simulink model "implementacao_em_blocos"  (R2013a)
settings: Solver=ode45  StartTime=0.0  StopTime=500  RelTol=1e-3
libraries: aerolibutil x4, vrlib x4, aerolibtransform2 x2, dspmtrx3 x1
settings Model: Creator=Daniel  LastModifiedBy=Daniel

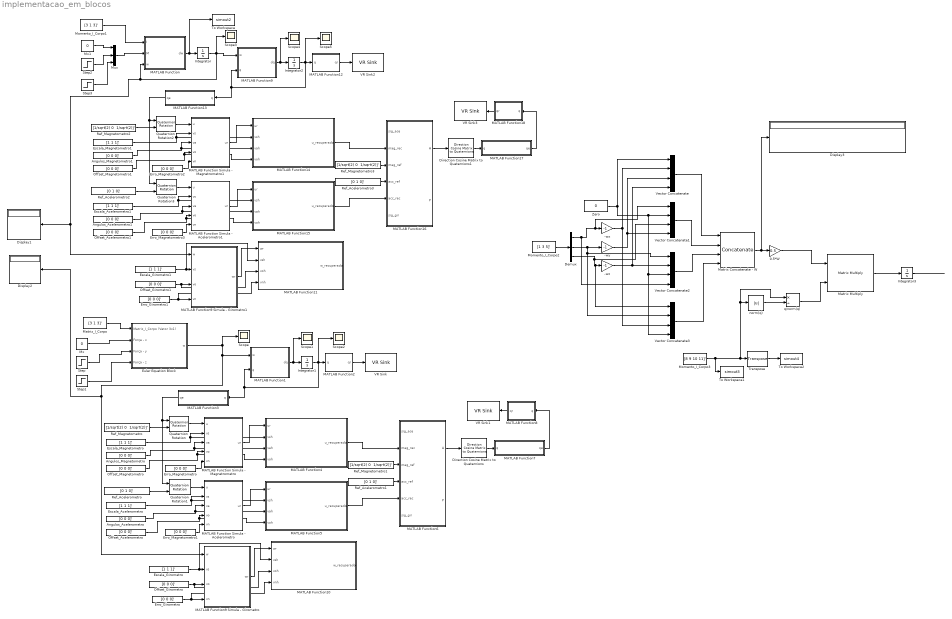
== system implementacao_em_blocos ==
  -wx : Gain  Gain=-1
  -wy : Gain  Gain=-1
  -wz : Gain  Gain=-1
  0.5*W : Gain  Gain=0.5
  Angulos_Acelerometro : Constant  Value=[0 0 0]'
  Angulos_Acelerometro1 : Constant  Value=[0 0 0]'
  Angulos_Magnetometro : Constant  Value=[0 0 0]'
  Angulos_Magnetometro1 : Constant  Value=[0 0 0]'
  Demux : Demux  Outputs=3
  Direction Cosine Matrix to Quaternions : aerolibtransform2/Direction Cosine Matrix  to Quaternions
  Direction Cosine Matrix to Quaternions1 : aerolibtransform2/Direction Cosine Matrix  to Quaternions
  Display1 : Display
  Display2 : Display
  Display3 : Display
  Erro_Girometro : Constant  Value=[0 0 0]'
  Erro_Girometro1 : Constant  Value=[0 0 0]'
  Erro_Magnetometro{,1..3} (4 alike) : Constant  Value=[0 0 0]'
  Escala_Acelerometro : Constant  Value=[1 1 1]'
  Escala_Acelerometro1 : Constant  Value=[1 1 1]'
  Escala_Girometro : Constant  Value=[1 1 1]'
  Escala_Girometro1 : Constant  Value=[1 1 1]'
  Escala_Magnetometro : Constant  Value=[1 1 1]'
  Escala_Magnetometro1 : Constant  Value=[1 1 1]'
  Euler Equation Block : Subsystem
  Integrator : Integrator  InitialCondition=[0 0 0]
  Integrator1 : Integrator  InitialCondition=[1 0 0 0]
  Integrator2 : Integrator  InitialCondition=[1 0 0 0]
  Integrator3 : Integrator  InitialCondition=[1 0 0 0]'
  MATLAB Function : MATLAB Function  TreatAsAtomicUnit=on
  MATLAB Function Simula - Acelerometro : MATLAB Function  TreatAsAtomicUnit=on
  MATLAB Function Simula - Acelerometro1 : MATLAB Function  TreatAsAtomicUnit=on
  MATLAB Function Simula - Magnetrometro : MATLAB Function  TreatAsAtomicUnit=on
  MATLAB Function Simula - Magnetrometro1 : MATLAB Function  TreatAsAtomicUnit=on
  MATLAB Function1 : MATLAB Function  TreatAsAtomicUnit=on
  MATLAB Function10 : MATLAB Function  TreatAsAtomicUnit=on
  MATLAB Function11 : MATLAB Function  TreatAsAtomicUnit=on
  MATLAB Function12 : MATLAB Function  TreatAsAtomicUnit=on
  MATLAB Function13 : MATLAB Function  TreatAsAtomicUnit=on
  MATLAB Function14 : MATLAB Function  TreatAsAtomicUnit=on
  MATLAB Function15 : MATLAB Function  TreatAsAtomicUnit=on
  MATLAB Function16 : MATLAB Function  TreatAsAtomicUnit=on
  MATLAB Function17 : MATLAB Function  TreatAsAtomicUnit=on
  MATLAB Function18 : MATLAB Function  TreatAsAtomicUnit=on
  MATLAB Function2 : MATLAB Function  TreatAsAtomicUnit=on
  MATLAB Function3 : MATLAB Function  TreatAsAtomicUnit=on
  MATLAB Function4 : MATLAB Function  TreatAsAtomicUnit=on
  MATLAB Function5 : MATLAB Function  TreatAsAtomicUnit=on
  MATLAB Function6 : MATLAB Function  TreatAsAtomicUnit=on
  MATLAB Function7 : MATLAB Function  TreatAsAtomicUnit=on
  MATLAB Function8 : MATLAB Function  TreatAsAtomicUnit=on
  MATLAB Function9 : MATLAB Function  TreatAsAtomicUnit=on
  MATLAB Function9 Simula - Girometro : MATLAB Function  TreatAsAtomicUnit=on
  MATLAB Function9 Simula - Girometro1 : MATLAB Function  TreatAsAtomicUnit=on
  Matrix Concatenate - W : Concatenate  NumInputs=4  Mode=Multidimensional array
  Matrix Multiply : Product  Multiplication=Matrix(*)
  Matriz_I_Corpo : Constant  Value=[3 1 3]'  VectorParams1D=off
  Momento_I_Corpo1 : Constant  Value=[3 1 3]'
  Momento_I_Corpo2 : Constant  Value=[1 3 5]'
  Momento_I_Corpo3 : Constant  Value=[8 9 10 11]'  VectorParams1D=off
  Mux : Mux  Inputs=3
  Mx : Constant  Value=0
  Mx1 : Constant  Value=0
  Offset_Acelerometro : Constant  Value=[0 0 0]'
  Offset_Acelerometro1 : Constant  Value=[0 0 0]'
  Offset_Girometro : Constant  Value=[0 0 0]'
  Offset_Girometro1 : Constant  Value=[0 0 0]'
  Offset_Magnetometro : Constant  Value=[0 0 0]'
  Offset_Magnetometro1 : Constant  Value=[0 0 0]'
  Quaternion Rotation{,1..3} (4 alike) : aerolibutil/Quaternion Rotation
  Ref_Acelerometro{,1..3} (4 alike) : Constant  Value=[0 1 0]'
  Ref_Magnetometro{,1..3} (4 alike) : Constant  Value="[1/sqrt(2) 0  1/sqrt(2)]'"
  Scope{,1..5} (6 alike) : Scope
      Scope2 settings: SaveName=ScopeData2
      Scope3 settings: SaveName=ScopeData3
      Scope4 settings: SaveName=ScopeData4
      Scope5 settings: SaveName=ScopeData5
  Step : Step  Before=1  After=0  SampleTime=0
  Step1 : Step  Before=.5  After=0  SampleTime=0
  Step2 : Step  Before=1  After=0  SampleTime=0
  Step3 : Step  Before=.5  After=0  SampleTime=0
  To Workspace : ToWorkspace  VariableName=simout2  SampleTime=-1
  To Workspace1 : ToWorkspace  VariableName=simout3  SampleTime=-1
  To Workspace2 : ToWorkspace  VariableName=simout4  SampleTime=-1
  Transpose : dspmtrx3/Transpose  Hermitian=off  overflowFlag=off
  VR Sink : vrlib/VR Sink  InstantiateOnLoad=on  SampleTime=.1  ViewEnable=on  RemoteChange=off  RemoteView=off  FieldsWritten=H.rotation.4.1.1.double  WorldFileName=C:\Users\Daniel\Desktop\TCC Daniel\Arquivos WRL\cilindro_bloco3.wrl  AutoView=off  VideoDimensions=[]  AllowVariableSize=off
  VR Sink1 : vrlib/VR Sink  InstantiateOnLoad=on  SampleTime=.1  ViewEnable=on  RemoteChange=off  RemoteView=off  FieldsWritten=H.rotation.4.1.1.double  WorldFileName=C:\Users\Daniel\Desktop\TCC Daniel\Arquivos WRL\cilindro_bloco4.wrl  AutoView=off  VideoDimensions=[]  AllowVariableSize=off
  VR Sink2 : vrlib/VR Sink  InstantiateOnLoad=on  SampleTime=.1  ViewEnable=on  RemoteChange=off  RemoteView=off  FieldsWritten=H.rotation.4.1.1.double  WorldFileName=C:\Users\Daniel\Desktop\TCC Daniel\Arquivos WRL\cilindro_bloco1.wrl  AutoView=off  VideoDimensions=[]  AllowVariableSize=off
  VR Sink3 : vrlib/VR Sink  InstantiateOnLoad=on  SampleTime=.1  ViewEnable=on  RemoteChange=off  RemoteView=off  FieldsWritten=H.rotation.4.1.1.double  WorldFileName=C:\Users\Daniel\Desktop\TCC Daniel\Arquivos WRL\cilindro_bloco2.wrl  AutoView=off  VideoDimensions=[]  AllowVariableSize=off
  Vector Concatenate{,1..3} (4 alike) : Concatenate  NumInputs=4  Mode=Multidimensional array  ConcatenateDimension=2
  Zero : Constant  Value=0
  norm(q) : Abs
  q/norm(q) : Product  Inputs=*/
  wires:
  Mux/1 -> MATLAB Function/2(M)
  MATLAB Function/1(dw) -> To Workspace/1, Integrator/1
  MATLAB Function1/1(dq) -> Integrator1/1, Scope1/1
  Integrator1/1 -> MATLAB Function3/1(q), MATLAB Function1/2(q), Scope2/1, MATLAB Function2/1(q)
  MATLAB Function2/1(qr) -> VR Sink/1
  Quaternion Rotation/1 -> MATLAB Function Simula - Magnetrometro/1(u)
  Quaternion Rotation1/1 -> MATLAB Function Simula - Acelerometro/1(u)
  MATLAB Function3/1(qe) -> Quaternion Rotation/1, Quaternion Rotation1/1
  Ref_Magnetometro/1 -> Quaternion Rotation/2
  Ref_Acelerometro/1 -> Quaternion Rotation1/2
  Erro_Magnetometro/1 -> MATLAB Function Simula - Magnetrometro/5(vn)
  Erro_Magnetometro1/1 -> MATLAB Function Simula - Acelerometro/5(vn)
  Offset_Magnetometro/1 -> MATLAB Function Simula - Magnetrometro/4(vo), MATLAB Function4/4(voh)
  Escala_Acelerometro/1 -> MATLAB Function Simula - Acelerometro/2(vs), MATLAB Function5/2(vsh)
  Angulos_Acelerometro/1 -> MATLAB Function Simula - Acelerometro/3(va), MATLAB Function5/3(vah)
  Offset_Acelerometro/1 -> MATLAB Function Simula - Acelerometro/4(vo), MATLAB Function5/4(voh)
  MATLAB Function Simula - Magnetrometro/1(ur) -> MATLAB Function4/1(ur)
  MATLAB Function Simula - Acelerometro/1(ur) -> MATLAB Function5/1(ur)
  Escala_Magnetometro/1 -> MATLAB Function Simula - Magnetrometro/2(vs), MATLAB Function4/2(vsh)
  Angulos_Magnetometro/1 -> MATLAB Function Simula - Magnetrometro/3(va), MATLAB Function4/3(vah)
  MATLAB Function5/1(u_recuperado) -> MATLAB Function6/5(acc_rec)
  MATLAB Function4/1(u_recuperado) -> MATLAB Function6/2(mag_rec)
  Ref_Magnetometro1/1 -> MATLAB Function6/3(mag_ref)
  Ref_Acelerometro1/1 -> MATLAB Function6/4(acc_ref)
  MATLAB Function6/1(A) -> Direction Cosine Matrix to Quaternions/1
  MATLAB Function7/1(qe) -> MATLAB Function8/1(q)
  MATLAB Function9 Simula - Girometro/1(wr) -> MATLAB Function10/1(wr)
  Escala_Girometro/1 -> MATLAB Function10/2(vsh), MATLAB Function9 Simula - Girometro/2(vs)
  Offset_Girometro/1 -> MATLAB Function10/3(voh), MATLAB Function9 Simula - Girometro/3(vo)
  Direction Cosine Matrix to Quaternions/1 -> MATLAB Function7/1(q)
  Erro_Girometro/1 -> MATLAB Function10/4(vnh), MATLAB Function9 Simula - Girometro/4(vn)
  MATLAB Function8/1(qr) -> VR Sink1/1
  MATLAB Function9/1(dq) -> Integrator2/1, Scope4/1
  Integrator2/1 -> MATLAB Function13/1(q), MATLAB Function9/2(q), Scope5/1, MATLAB Function12/1(q)
  MATLAB Function12/1(qr) -> VR Sink2/1
  Quaternion Rotation2/1 -> MATLAB Function Simula - Magnetrometro1/1(u)
  Quaternion Rotation3/1 -> MATLAB Function Simula - Acelerometro1/1(u)
  MATLAB Function13/1(qe) -> Quaternion Rotation2/1, Quaternion Rotation3/1
  Ref_Magnetometro2/1 -> Quaternion Rotation2/2
  Ref_Acelerometro2/1 -> Quaternion Rotation3/2
  Erro_Magnetometro2/1 -> MATLAB Function Simula - Magnetrometro1/5(vn)
  Erro_Magnetometro3/1 -> MATLAB Function Simula - Acelerometro1/5(vn)
  Offset_Magnetometro1/1 -> MATLAB Function Simula - Magnetrometro1/4(vo), MATLAB Function14/4(voh)
  Escala_Acelerometro1/1 -> MATLAB Function Simula - Acelerometro1/2(vs), MATLAB Function15/2(vsh)
  Angulos_Acelerometro1/1 -> MATLAB Function Simula - Acelerometro1/3(va), MATLAB Function15/3(vah)
  Offset_Acelerometro1/1 -> MATLAB Function Simula - Acelerometro1/4(vo), MATLAB Function15/4(voh)
  MATLAB Function Simula - Magnetrometro1/1(ur) -> MATLAB Function14/1(ur)
  MATLAB Function Simula - Acelerometro1/1(ur) -> MATLAB Function15/1(ur)
  Escala_Magnetometro1/1 -> MATLAB Function Simula - Magnetrometro1/2(vs), MATLAB Function14/2(vsh)
  Angulos_Magnetometro1/1 -> MATLAB Function Simula - Magnetrometro1/3(va), MATLAB Function14/3(vah)
  MATLAB Function15/1(u_recuperado) -> MATLAB Function16/5(acc_rec)
  MATLAB Function14/1(u_recuperado) -> MATLAB Function16/2(mag_rec)
  Ref_Magnetometro3/1 -> MATLAB Function16/3(mag_ref)
  Ref_Acelerometro3/1 -> MATLAB Function16/4(acc_ref)
  MATLAB Function16/1(A) -> Direction Cosine Matrix to Quaternions1/1
  MATLAB Function17/1(qe) -> MATLAB Function18/1(q)
  MATLAB Function9 Simula - Girometro1/1(wr) -> MATLAB Function11/1(wr)
  Escala_Girometro1/1 -> MATLAB Function11/2(vsh), MATLAB Function9 Simula - Girometro1/2(vs)
  Offset_Girometro1/1 -> MATLAB Function11/3(voh), MATLAB Function9 Simula - Girometro1/3(vo)
  Direction Cosine Matrix to Quaternions1/1 -> MATLAB Function17/1(q)
  Erro_Girometro1/1 -> MATLAB Function11/4(vnh), MATLAB Function9 Simula - Girometro1/4(vn)
  MATLAB Function18/1(qr) -> VR Sink3/1
  Matriz_I_Corpo/1 -> Euler Equation Block/1(Matriz_I_Corpo (Vetor 3x1))
  Mx/1 -> Euler Equation Block/2(Força - x)
  Step/1 -> Euler Equation Block/3(Força - y)
  Step1/1 -> Euler Equation Block/4(Força - z)
  Momento_I_Corpo1/1 -> MATLAB Function/1(I)
  Mx1/1 -> Mux/1
  Step2/1 -> Mux/2
  Step3/1 -> Mux/3
  Integrator/1 -> Scope3/1, MATLAB Function/3(w), Display1/1, MATLAB Function9 Simula - Girometro1/1(w), MATLAB Function9/1(w)
  Euler Equation Block/1(w) -> MATLAB Function9 Simula - Girometro/1(w), Display2/1, MATLAB Function1/1(w), Scope/1
  Momento_I_Corpo3/1 -> To Workspace1/1, Transpose/1, q/norm(q)/1, norm(q)/1
  norm(q)/1 -> q/norm(q)/2
  Demux/3 -> Vector Concatenate3/1, -wz/1, Vector Concatenate1/3
  Demux/2 -> Vector Concatenate3/2, Vector Concatenate2/1, -wy/1
  Demux/1 -> Vector Concatenate2/4, Vector Concatenate1/1, -wx/1
  Zero/1 -> Vector Concatenate3/4, Vector Concatenate2/3, Vector Concatenate1/2, Vector Concatenate/1
  -wx/1 -> Vector Concatenate3/3, Vector Concatenate/2
  -wy/1 -> Vector Concatenate1/4, Vector Concatenate/3
  -wz/1 -> Vector Concatenate2/2, Vector Concatenate/4
  Vector Concatenate/1 -> Matrix Concatenate - W/1
  Vector Concatenate1/1 -> Matrix Concatenate - W/2
  Vector Concatenate2/1 -> Matrix Concatenate - W/3
  Vector Concatenate3/1 -> Matrix Concatenate - W/4
  Matrix Concatenate - W/1 -> 0.5*W/1, Display3/1
  Momento_I_Corpo2/1 -> Demux/1
  q/norm(q)/1 -> Matrix Multiply/2
  0.5*W/1 -> Matrix Multiply/1
  Transpose/1 -> To Workspace2/1
  Matrix Multiply/1 -> Integrator3/1
  Integrator3/1 -> ?

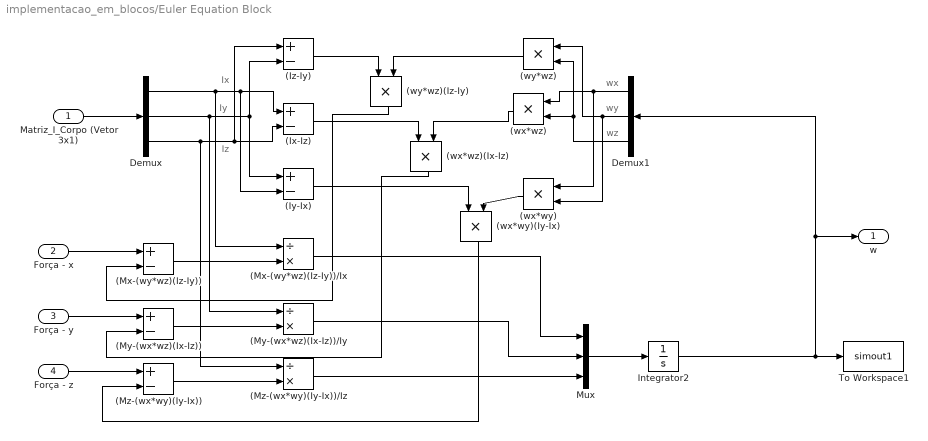
== system implementacao_em_blocos/Euler Equation Block ==
  note: Iz
  note: Iy
  note: Ix
  note: wy
  note: wx
  note: wz
  Matriz_I_Corpo (Vetor 3x1) : Inport
  Força - x : Inport  Port=2
  Força - y : Inport  Port=3
  Força - z : Inport  Port=4
  (Ix-Iz) : Sum  Inputs=+-
  (Iy-Ix) : Sum  Inputs=+-
  (Iz-Iy) : Sum  Inputs=+-
  (Mx-(wy*wz)(Iz-Iy)) : Sum  Inputs=+-
  (Mx-(wy*wz)(Iz-Iy))/Ix : Product  Inputs=/*
  (My-(wx*wz)(Ix-Iz)) : Sum  Inputs=+-
  (My-(wx*wz)(Ix-Iz))/Iy : Product  Inputs=/*
  (Mz-(wx*wy)(Iy-Ix)) : Sum  Inputs=+-
  (Mz-(wx*wy)(Iy-Ix))/Iz : Product  Inputs=/*
  (wx*wy) : Product
  (wx*wy)(Iy-Ix) : Product
  (wx*wz) : Product
  (wx*wz)(Ix-Iz) : Product
  (wy*wz) : Product
  (wy*wz)(Iz-Iy) : Product
  Demux : Demux  Outputs=3
  Demux1 : Demux  Outputs=3
  Integrator2 : Integrator  InitialCondition=[0 0 0]
  Mux : Mux  Inputs=3
  To Workspace1 : ToWorkspace  VariableName=simout1  SampleTime=-1
  w : Outport
  wires:
  (Mz-(wx*wy)(Iy-Ix))/1 -> (Mz-(wx*wy)(Iy-Ix))/Iz/2
  Demux/3 -> (Mz-(wx*wy)(Iy-Ix))/Iz/1, (Iz-Iy)/1, (Ix-Iz)/2
  Força - z/1 -> (Mz-(wx*wy)(Iy-Ix))/1
  (wx*wy)(Iy-Ix)/1 -> (Mz-(wx*wy)(Iy-Ix))/2
  (wy*wz)(Iz-Iy)/1 -> (Mx-(wy*wz)(Iz-Iy))/2
  (My-(wx*wz)(Ix-Iz))/1 -> (My-(wx*wz)(Ix-Iz))/Iy/2
  (My-(wx*wz)(Ix-Iz))/Iy/1 -> Mux/2
  (Iz-Iy)/1 -> (wy*wz)(Iz-Iy)/1
  Demux1/2 -> (wx*wy)/2, (wy*wz)/1
  (Ix-Iz)/1 -> (wx*wz)(Ix-Iz)/1
  (wx*wz)/1 -> (wx*wz)(Ix-Iz)/2
  (wy*wz)/1 -> (wy*wz)(Iz-Iy)/2
  Demux1/1 -> (wx*wy)/1, (wx*wz)/1
  Demux1/3 -> (wy*wz)/2, (wx*wz)/2
  (wx*wy)/1 -> (wx*wy)(Iy-Ix)/2
  (Iy-Ix)/1 -> (wx*wy)(Iy-Ix)/1
  (wx*wz)(Ix-Iz)/1 -> (My-(wx*wz)(Ix-Iz))/2
  Força - x/1 -> (Mx-(wy*wz)(Iz-Iy))/1
  (Mz-(wx*wy)(Iy-Ix))/Iz/1 -> Mux/3
  Demux/1 -> (Mx-(wy*wz)(Iz-Iy))/Ix/1, (Iy-Ix)/2, (Ix-Iz)/1
  Demux/2 -> (My-(wx*wz)(Ix-Iz))/Iy/1, (Iy-Ix)/1, (Iz-Iy)/2
  (Mx-(wy*wz)(Iz-Iy))/1 -> (Mx-(wy*wz)(Iz-Iy))/Ix/2
  Força - y/1 -> (My-(wx*wz)(Ix-Iz))/1
  Matriz_I_Corpo (Vetor 3x1)/1 -> Demux/1
  Mux/1 -> Integrator2/1
  (Mx-(wy*wz)(Iz-Iy))/Ix/1 -> Mux/1
  Integrator2/1 -> To Workspace1/1, Demux1/1, w/1

== matlab function implementacao_em_blocos/MATLAB Function1 ==
  data: w input; dq output; q input
function dq = cinematica(w,q)
%#eml
wx = w(1);
wy = w(2);
wz = w(3);

q = q/norm(q);

qteta = q(1);
qx = q(2);
qy = q(3);
qz = q(4);

W = [0 -wx -wy -wz; wx 0 wz -wy; wy -wz 0 wx; wz wy -wx 0];
%W=[0 wz -wy wx; -wz 0 wx wy; wy -wx 0 wz; -wx -wy -wz 0];
dq=0.5*W*[qteta qx qy qz]';

== matlab function implementacao_em_blocos/MATLAB Function ==
  data: I input; dw output; M input; w input
function dw  = Eq_Euler(I,M,w)
%#eml
wx = w(1);
wy = w(2);
wz = w(3);

Ix = I(1);
Iy = I(2);
Iz = I(3);

Mx = M(1);
My = M(2);
Mz = M(3);

dwx = (Mx - wy*wz*(Iz - Iy))/Ix;
dwy = (My - wx*wz*(Ix - Iz))/Iy;
dwz = (Mz - wx*wy*(Iy - Ix))/Iz;

dw=[dwx dwy dwz];

== matlab function implementacao_em_blocos/MATLAB Function2 ==
  data: q input; qr output
function qr = ajusta_q(q)
%#eml

q = q/(norm(q));
v = [q(2) q(3) q(4)] / norm([q(2) q(3) q(4)]);
ang = acos(q(1))*2;

qr = [v ang];

== matlab function implementacao_em_blocos/MATLAB Function3 ==
  data: q input; qe output
function qe = tira_redundancia(q)
qe = zeros(4,1);
%#eml

if q(1)<0
    qe = -q;
else
    qe = q;
end

== matlab function implementacao_em_blocos/MATLAB Function Simula - Magnetrometro ==
  data: u input; ur output; vs input; va input; vo input; vn input
function ur = triad_model(u,vs,va,vo,vn)
%#eml

rho = va(1);
phi = va(2);
lambda = va(3);

S = diag(vs);
T = [1 0 0; sin(rho) cos(rho) 0;...
    sin(phi)*cos(lambda) sin(lambda)*cos(phi) cos(phi)*cos(lambda)];

ur = S*T*u + vo + vn*randn;

== matlab function implementacao_em_blocos/MATLAB Function Simula - Acelerometro ==
  data: u input; ur output; vs input; va input; vo input; vn input
function ur = triad_model(u,vs,va,vo,vn)
%#eml

rho = va(1);
phi = va(2);
lambda = va(3);

S = diag(vs);
T = [1 0 0; sin(rho) cos(rho) 0;...
    sin(phi)*cos(lambda) sin(lambda)*cos(phi) cos(phi)*cos(lambda)];

ur = S*T*u + vo + vn*randn;

== matlab function implementacao_em_blocos/MATLAB Function4 ==
  data: ur input; u_recuperado output; vsh input; vah input; voh input
function u_recuperado = inv_triad_model(ur,vsh,vah,voh)
%#eml

rho = vah(1);
phi = vah(2);
lambda = vah(3);

T_inv = [1 0 0; -tan(rho) 1/cos(rho) 0;...
    tan(rho)*tan(lambda)-tan(phi) -tan(lambda)/cos(rho) 1/(cos(lambda)*cos(phi))];
S_inv = inv(diag(vsh));

u_recuperado = T_inv*S_inv*(ur - voh);

== matlab function implementacao_em_blocos/MATLAB Function5 ==
  data: ur input; u_recuperado output; vsh input; vah input; voh input
function u_recuperado = inv_triad_model(ur,vsh,vah,voh)
%#eml

rho = vah(1);
phi = vah(2);
lambda = vah(3);

T_inv = [1 0 0; -tan(rho) 1/cos(rho) 0;...
    tan(rho)*tan(lambda)-tan(phi) -tan(lambda)/cos(rho) 1/(cos(lambda)*cos(phi))];
S_inv = inv(diag(vsh));

u_recuperado = T_inv*S_inv*(ur - voh);

== matlab function implementacao_em_blocos/MATLAB Function6 ==
  data: sig_ace input; A output; mag_rec input; mag_ref input; acc_ref input; acc_rec input; sig_gir input; P output
function [A,P] = TRIAD(sig_ace,mag_rec,mag_ref,acc_ref,acc_rec,sig_gir)

% ========== Função de Determinação de Atitude ===========
% ========== Algoritmo TRIAD ===========
% Os parâmetros de Entrada são:
% V1 : vetor de referência V1
V1 = acc_ref;
% V2 : vetor de referência V2
V2 = mag_ref;
% W1 : vetor de observação W1
W1 = acc_rec;
% W2 : vetor de observação W2
W2 = mag_rec;
% SigTo1 : desvio padrão das observação do Acelerômetro
SigTot1 = sig_ace;
% SigTo2 : desvio padrão das observação do Magnetômetro
SigTot2 = sig_gir;

% ========================================================
% Os parâmetros de Retorno são:
% A : matriz de atitude
% P : Covariância da atitude
% ========================================================
% --- Obtendo a Tríade de Referência
r1 = V1/norm(V1);
r2 = cross(V1,V2); % função do produto vetorial
r2 = r2 / norm(r2);
r3 = cross(r1,r2);
% --- Montando a Matriz de Referência
Mref = [r1 r2 r3];
% --- Obtendo a tríade de observação
s1 = W1/norm(W1);
s2 = cross(W1,W2);
s2 = s2 / norm(s2);
s3 = cross(s1,s2);
% --- Montando a Matriz de Observação
Mobs = [s1 s2 s3];
% --- Atitude pelo TRIAD
A = Mobs * Mref';
%--------------------------------------------------------------------------
% Obtendo a covariância da atitude (P = P + AP AT)
P = SigTot1^2 * eye(3) + ...
    (1/norm(cross(W1,W2)))^2 * (SigTot1^2* (W1'*W2) * (W1*W2' + W2*W1')...
    + (SigTot2^2 - SigTot1^2)*W1*W1');

%--------------------------------------------------------------------------

== matlab function implementacao_em_blocos/MATLAB Function7 ==
  data: q input; qe output
function qe = tira_redundancia(q)
qe = zeros(4,1);
%#eml

if q(1)<0
    qe = -q;
else
    qe = q;
end

== matlab function implementacao_em_blocos/MATLAB Function8 ==
  data: q input; qr output
function qr = ajusta_q(q)
%#eml

q = q/(norm(q));
v = [q(2) q(3) q(4)] / norm([q(2) q(3) q(4)]);
ang = acos(q(1))*2;

qr = [v ang];

== matlab function implementacao_em_blocos/MATLAB Function9 Simula - Girometro ==
  data: w input; wr output; vs input; vo input; vn input
function wr = gyro_model(w,vs,vo,vn)
%#eml

S = diag(vs);

wr = S*w + vo + vn*randn;

== matlab function implementacao_em_blocos/MATLAB Function10 ==
  data: wr input; w_recuperado output; vsh input; voh input; vnh input
function w_recuperado = inv_gyro_model(wr,vsh,voh,vnh)
%#eml

S_inv = inv(diag(vsh));

w_recuperado = S_inv*(wr - voh);

== matlab function implementacao_em_blocos/MATLAB Function Simula - Acelerometro1 ==
  data: u input; ur output; vs input; va input; vo input; vn input
function ur = triad_model(u,vs,va,vo,vn)
%#eml

rho = va(1);
phi = va(2);
lambda = va(3);

S = diag(vs);
T = [1 0 0; sin(rho) cos(rho) 0;...
    sin(phi)*cos(lambda) sin(lambda)*cos(phi) cos(phi)*cos(lambda)];

ur = S*T*u + vo + vn*randn;

== matlab function implementacao_em_blocos/MATLAB Function Simula - Magnetrometro1 ==
  data: u input; ur output; vs input; va input; vo input; vn input
function ur = triad_model(u,vs,va,vo,vn)
%#eml

rho = va(1);
phi = va(2);
lambda = va(3);

S = diag(vs);
T = [1 0 0; sin(rho) cos(rho) 0;...
    sin(phi)*cos(lambda) sin(lambda)*cos(phi) cos(phi)*cos(lambda)];

ur = S*T*u + vo + vn*randn;

== matlab function implementacao_em_blocos/MATLAB Function11 ==
  data: wr input; w_recuperado output; vsh input; voh input; vnh input
function w_recuperado = inv_gyro_model(wr,vsh,voh,vnh)
%#eml

S_inv = inv(diag(vsh));

w_recuperado = S_inv*(wr - voh);

== matlab function implementacao_em_blocos/MATLAB Function12 ==
  data: q input; qr output
function qr = ajusta_q(q)
%#eml

q = q/(norm(q));
v = [q(2) q(3) q(4)] / norm([q(2) q(3) q(4)]);
ang = acos(q(1))*2;

qr = [v ang];

== matlab function implementacao_em_blocos/MATLAB Function13 ==
  data: q input; qe output
function qe = tira_redundancia(q)
qe = zeros(4,1);
%#eml

if q(1)<0
    qe = -q;
else
    qe = q;
end

== matlab function implementacao_em_blocos/MATLAB Function14 ==
  data: ur input; u_recuperado output; vsh input; vah input; voh input
function u_recuperado = inv_triad_model(ur,vsh,vah,voh)
%#eml

rho = vah(1);
phi = vah(2);
lambda = vah(3);

T_inv = [1 0 0; -tan(rho) 1/cos(rho) 0;...
    tan(rho)*tan(lambda)-tan(phi) -tan(lambda)/cos(rho) 1/(cos(lambda)*cos(phi))];
S_inv = inv(diag(vsh));

u_recuperado = T_inv*S_inv*(ur - voh);

== matlab function implementacao_em_blocos/MATLAB Function15 ==
  data: ur input; u_recuperado output; vsh input; vah input; voh input
function u_recuperado = inv_triad_model(ur,vsh,vah,voh)
%#eml

rho = vah(1);
phi = vah(2);
lambda = vah(3);

T_inv = [1 0 0; -tan(rho) 1/cos(rho) 0;...
    tan(rho)*tan(lambda)-tan(phi) -tan(lambda)/cos(rho) 1/(cos(lambda)*cos(phi))];
S_inv = inv(diag(vsh));

u_recuperado = T_inv*S_inv*(ur - voh);

== matlab function implementacao_em_blocos/MATLAB Function16 ==
  data: sig_ace input; A output; mag_rec input; mag_ref input; acc_ref input; acc_rec input; sig_gir input; P output
function [A,P] = TRIAD(sig_ace,mag_rec,mag_ref,acc_ref,acc_rec,sig_gir)

% ========== Função de Determinação de Atitude ===========
% ========== Algoritmo TRIAD ===========
% Os parâmetros de Entrada são:
% V1 : vetor de referência V1
V1 = acc_ref;
% V2 : vetor de referência V2
V2 = mag_ref;
% W1 : vetor de observação W1
W1 = acc_rec;
% W2 : vetor de observação W2
W2 = mag_rec;
% SigTo1 : desvio padrão das observação do Acelerômetro
SigTot1 = sig_ace;
% SigTo2 : desvio padrão das observação do Magnetômetro
SigTot2 = sig_gir;

% ========================================================
% Os parâmetros de Retorno são:
% A : matriz de atitude
% P : Covariância da atitude
% ========================================================
% --- Obtendo a Tríade de Referência
r1 = V1/norm(V1);
r2 = cross(V1,V2); % função do produto vetorial
r2 = r2 / norm(r2);
r3 = cross(r1,r2);
% --- Montando a Matriz de Referência
Mref = [r1 r2 r3];
% --- Obtendo a tríade de observação
s1 = W1/norm(W1);
s2 = cross(W1,W2);
s2 = s2 / norm(s2);
s3 = cross(s1,s2);
% --- Montando a Matriz de Observação
Mobs = [s1 s2 s3];
% --- Atitude pelo TRIAD
A = Mobs * Mref';
%--------------------------------------------------------------------------
% Obtendo a covariância da atitude (P = P + AP AT)
P = SigTot1^2 * eye(3) + ...
    (1/norm(cross(W1,W2)))^2 * (SigTot1^2* (W1'*W2) * (W1*W2' + W2*W1')...
    + (SigTot2^2 - SigTot1^2)*W1*W1');

%--------------------------------------------------------------------------

== matlab function implementacao_em_blocos/MATLAB Function17 ==
  data: q input; qe output
function qe = tira_redundancia(q)
qe = zeros(4,1);
%#eml

if q(1)<0
    qe = -q;
else
    qe = q;
end

== matlab function implementacao_em_blocos/MATLAB Function18 ==
  data: q input; qr output
function qr = ajusta_q(q)
%#eml

q = q/(norm(q));
v = [q(2) q(3) q(4)] / norm([q(2) q(3) q(4)]);
ang = acos(q(1))*2;

qr = [v ang];

== matlab function implementacao_em_blocos/MATLAB Function9 ==
  data: w input; dq output; q input
function dq = cinematica(w,q)
%#eml
wx = w(1);
wy = w(2);
wz = w(3);

q = q/norm(q);

qteta = q(1);
qx = q(2);
qy = q(3);
qz = q(4);

W = [0 -wx -wy -wz; wx 0 wz -wy; wy -wz 0 wx; wz wy -wx 0];
%W=[0 wz -wy wx; -wz 0 wx wy; wy -wx 0 wz; -wx -wy -wz 0];
dq=0.5*W*[qteta qx qy qz]';

== matlab function implementacao_em_blocos/MATLAB Function9 Simula - Girometro1 ==
  data: w input; wr output; vs input; vo input; vn input
function wr = gyro_model(w,vs,vo,vn)
%#eml

S = diag(vs);

wr = S*w + vo + vn*randn;
